simulink model "Kalman_State_space"  (R2013a)
settings: Solver=ode45  StartTime=0.0  StopTime=10.0  RelTol=1e-3
values from neighbouring files (symbols this model uses):
  K = sigma * A*P*inv(s)    [Brid_code.m]    (also in Kalman_Filter.m = A_d*P*inv(s))
undefined symbols (not defined in the file or in its folder): F, H
settings Model: Creator=user  LastModifiedBy=user

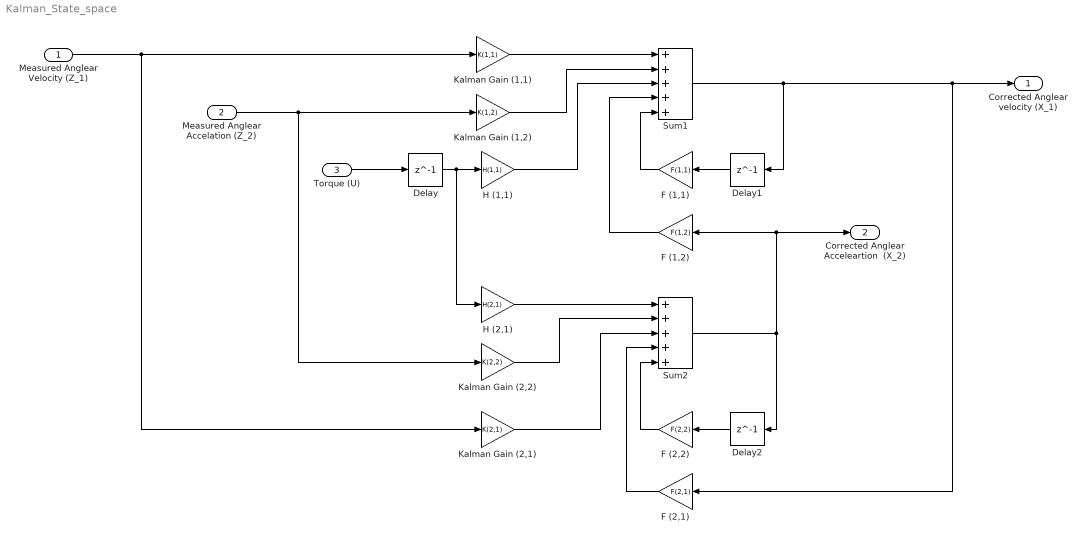
== system Kalman_State_space ==
  "Measured Anglear Velocity (Z_1) " : Inport
  Measured Anglear Accelation (Z_2) : Inport  Port=2
  Torque (U) : Inport  Port=3
  Delay : Delay  DelayLength=1  InitialCondition=0
  Delay1 : Delay  DelayLength=1  InitialCondition=0
  Delay2 : Delay  DelayLength=1  InitialCondition=0
  F (1,1) : Gain  Gain=F(1,1)
  F (1,2) : Gain  Gain=F(1,2)
  F (2,1) : Gain  Gain=F(2,1)
  F (2,2) : Gain  Gain=F(2,2)
  H (1,1) : Gain  Gain=H(1,1)
  H (2,1) : Gain  Gain=H(2,1)
  Kalman Gain (1,1) : Gain  Gain=K(1,1)
  Kalman Gain (1,2) : Gain  Gain=K(1,2)
  Kalman Gain (2,1) : Gain  Gain=K(2,1)
  Kalman Gain (2,2) : Gain  Gain=K(2,2)
  Sum1 : Sum  Inputs=+++++
  Sum2 : Sum  Inputs=+++++
  Corrected Anglear velocity (X_1) : Outport
  Corrected Anglear Acceleartion  (X_2) : Outport  Port=2
  wires:
  Kalman Gain (1,1)/1 -> Sum1/1
  Kalman Gain (1,2)/1 -> Sum1/2
  H (1,1)/1 -> Sum1/3
  Sum1/1 -> Corrected Anglear velocity (X_1)/1, F (2,1)/1, Delay1/1
  Delay1/1 -> F (1,1)/1
  F (1,1)/1 -> Sum1/5
  H (2,1)/1 -> Sum2/1
  Kalman Gain (2,2)/1 -> Sum2/2
  Kalman Gain (2,1)/1 -> Sum2/3
  Delay2/1 -> F (2,2)/1
  F (2,2)/1 -> Sum2/5
  Delay/1 -> H (2,1)/1, H (1,1)/1
  "Measured Anglear Velocity (Z_1) "/1 -> Kalman Gain (1,1)/1, Kalman Gain (2,1)/1
  Measured Anglear Accelation (Z_2)/1 -> Kalman Gain (2,2)/1, Kalman Gain (1,2)/1
  Torque (U)/1 -> Delay/1
  F (1,2)/1 -> Sum1/4
  F (2,1)/1 -> Sum2/4
  Sum2/1 -> Corrected Anglear Acceleartion  (X_2)/1, F (1,2)/1, Delay2/1
